simulink model "Threephase_PWM_Inverter"  (R2022b)
settings: Solver=VariableStepAuto  StartTime=0.0  StopTime=2  MaxStep=1e-6
InitFcn:
  | fs=20e3;
  | Ts=1/fs;
  | Udc=700;
  | Cf=20e-6;
  | Rf=0.1;
  | Lf=3e-3;
  | Rg=0.2;
  | Lg=4e-3;
  | wCf=100*pi*Cf;
  | wLf=100*pi*Lf;
  | 
  | Vn=220*sqrt(2);
  | Qn=5000;
  | wn=2*pi*50;
  | Pn=20e3;
  | m=0.01*wn/Pn;
  | kw=1/m;
  | n=1/20*Vn/Qn;
  | J=0.5; %0.2 0.5 0.8
  | D=20;%D=5 10
  | 
  | kp_v=3; %3
  | ki_v=8; %8
  | kp_i=95; %95
  | ki_i=100; %100
libraries: simulink x7, spsabctodq0Lib x6, slpidlib x5, spsThreePhaseSeriesRLCLoadLib x4, spsThreePhaseVIMeasurementLib x4, spsPower3phInstantaneousLib x3, spsThreePhaseBreakerLib x3, spsPLL3phLib x2, spsThreePhaseSeriesRLCBranchLib x2, spsDCVoltageSourceLib x1, spsGroundLib x1, spsUniversalBridgeLib x1
settings Model: Creator=Administrator  LastModifiedBy=Zeren
settings SolverCC: AlgebraicLoopSolver=TrustRegion
settings DataIOCC: ReturnWorkspaceOutputs=off
settings DebuggingCC: UnconnectedInputMsg=warning  UnconnectedOutputMsg=warning  UnconnectedLineMsg=warning  SFMachineParentedDataDiag=warning  ArithmeticOperatorsInVariantConditions=warning
settings ModelReferenceCC: EnableRefExpFcnMdlSchedulingChecks=on
settings SFSimCC: SimUseLocalCustomCode=off  CustomCodeUndefinedFunction=UseInterfaceOnly
settings RTWCC: RTWUseLocalCustomCode=off

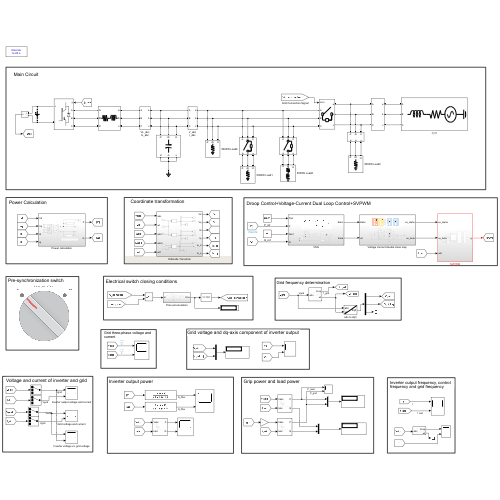
[thumbnail: Simulink's stored preview of the top-level diagram]
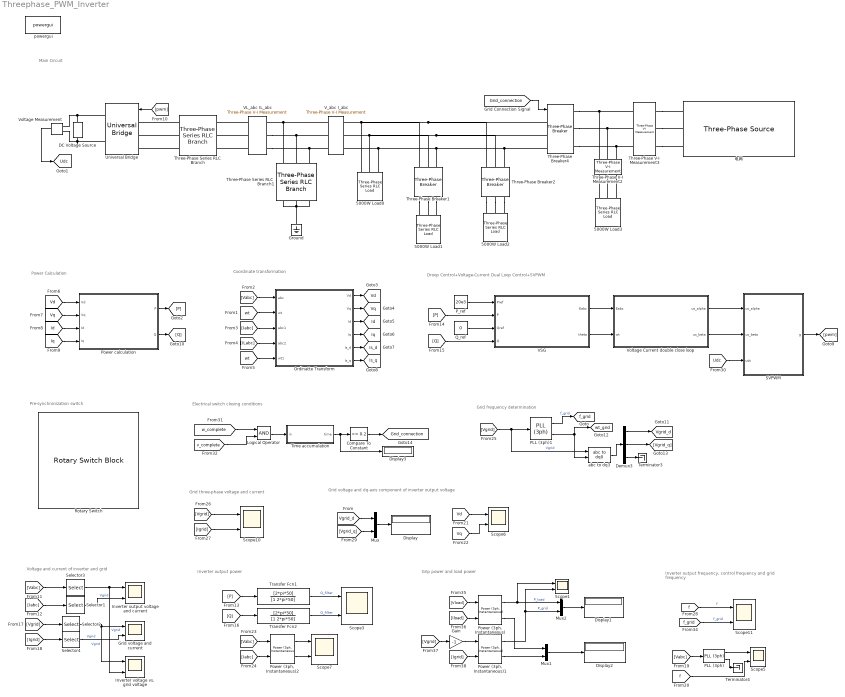
== system Threephase_PWM_Inverter ==
  note: Grid voltage and dq-axis component of inverter output voltage
  note: Grip power and load power
  note: Grid three-phase voltage and current
  note: Voltage and current of inverter and grid
  note: Inverter output frequency, control frequency and grid frequency
  note: Inverter output power
  note: Main Circuit
  note: Grid frequency determination
  note: Power Calculation
  note: Electrical switch closing conditions
  note: Pre-synchronization switch
  note: Coordinate transformation
  note: Droop Control+Voltage-Current Dual Loop Control+SVPWM
  5000W Load0 : spsThreePhaseSeriesRLCLoadLib/Three-Phase Series RLC Load  LConnTagsString=A|B|C  Configuration=Y (grounded)  NominalVoltage=380  Vabc=[1e3 1e3 1e3]  Vabcp=[1e3 1e3 1e3]  NominalFrequency=50  UnbalancedPower=off  ActivePower=5e3  InductivePower=0  CapacitivePower=0  Pabc=[10e3 9e3 11e3]  QLabc=[100 90 110]  QCabc=[100 90 110]  Pabcp=[10e3 9e3 11e3]  QLabcp=[100 90 110]  QCabcp=[100 90 110]  Measurements=None  LoadType=constant Z
  5000W Load1 : spsThreePhaseSeriesRLCLoadLib/Three-Phase Series RLC Load  LConnTagsString=A|B|C  Configuration=Y (grounded)  NominalVoltage=380  Vabc=[1e3 1e3 1e3]  Vabcp=[1e3 1e3 1e3]  NominalFrequency=50  UnbalancedPower=off  ActivePower=5e3  InductivePower=0  CapacitivePower=0  Pabc=[10e3 9e3 11e3]  QLabc=[100 90 110]  QCabc=[100 90 110]  Pabcp=[10e3 9e3 11e3]  QLabcp=[100 90 110]  QCabcp=[100 90 110]  Measurements=None  LoadType=constant Z
  5000W Load2 : spsThreePhaseSeriesRLCLoadLib/Three-Phase Series RLC Load  LConnTagsString=A|B|C  Configuration=Y (grounded)  NominalVoltage=380  Vabc=[1e3 1e3 1e3]  Vabcp=[1e3 1e3 1e3]  NominalFrequency=50  UnbalancedPower=off  ActivePower=5e3  InductivePower=500  CapacitivePower=0  Pabc=[10e3 9e3 11e3]  QLabc=[100 90 110]  QCabc=[100 90 110]  Pabcp=[10e3 9e3 11e3]  QLabcp=[100 90 110]  QCabcp=[100 90 110]  Measurements=None  LoadType=constant Z
  5000W Load3 : spsThreePhaseSeriesRLCLoadLib/Three-Phase Series RLC Load  LConnTagsString=A|B|C  Configuration=Y (grounded)  NominalVoltage=380  Vabc=[1e3 1e3 1e3]  Vabcp=[1e3 1e3 1e3]  NominalFrequency=50  UnbalancedPower=off  ActivePower=5e3  InductivePower=0  CapacitivePower=0  Pabc=[10e3 9e3 11e3]  QLabc=[100 90 110]  QCabc=[100 90 110]  Pabcp=[10e3 9e3 11e3]  QLabcp=[100 90 110]  QCabcp=[100 90 110]  Measurements=None  LoadType=constant Z
  Compare To Constant : simulink/Logic and Bit Operations/Compare To Constant  relop=>=  const=0.2  OutDataTypeStr=boolean
  DC Voltage Source : spsDCVoltageSourceLib/DC Voltage Source  Amplitude=800  Measurements=None
  Demux3 : Demux  Outputs=3
  Display{,1..3} (4 alike) : Display
  Gain : Gain  Gain=-1
  Grid voltage and current : Scope  NumInputPorts=2
  Ground : spsGroundLib/Ground  LConnTagsString=a
  Inverter output voltage and current : Scope  NumInputPorts=2
  Inverter voltage vs. grid voltage : Scope  NumInputPorts=2
  Logical Operator : Logic  AllPortsSameDT=off  OutDataTypeStr=boolean
  Mux : Mux  Inputs=2
  Mux1 : Mux  Inputs=2
  Mux2 : Mux  Inputs=2
  Ordinatte Transform : Subsystem
  PLL (3ph) : spsPLL3phLib/PLL (3ph)  Fmin=45  Par_Init=[0, 50]  ParK=[180, 3200, 1]  TcD=1e-4  MaxRateChangeFreq=12  FilterCutOffFreq=25  Ts=0  AGC=on
  PLL (3ph)1 : spsPLL3phLib/PLL (3ph)  Fmin=45  Par_Init=[0, 50]  ParK=[180, 3200, 1]  TcD=1e-4  MaxRateChangeFreq=12  FilterCutOffFreq=25  Ts=0  AGC=on
  P_ref : Constant  Value=20e3
  "Power (3ph, Instantaneous)" : spsPower3phInstantaneousLib/Power (3ph, Instantaneous)
  "Power (3ph, Instantaneous)1" : spsPower3phInstantaneousLib/Power (3ph, Instantaneous)
  "Power (3ph, Instantaneous)2" : spsPower3phInstantaneousLib/Power (3ph, Instantaneous)
  Power calculation : Subsystem
  Q_ref : Constant  Value=0
  Rotary Switch : RotarySwitchBlock
      settings: Values={{'Off', 'On'}, [0 1]}
  SVPWM : Subsystem
  Scope{1,3,5..7,10..11} (7 alike) : Scope  NumInputPorts=2
  Selector{1..4} (4 alike) : Selector  InputPortWidth=3  IndexOptions=Index vector (dialog)  Indices=[1]  OutputSizes=1
  Terminator3 : Terminator
  Terminator4 : Terminator
  Three-Phase Series RLC Branch : spsThreePhaseSeriesRLCBranchLib/Three-Phase Series RLC Branch  LConnTagsString=A|B|C  RConnTagsString=A|B|C  BranchType=RL  Resistance=1e-4  Inductance=5e-3  Capacitance=1e-6  Measurements=None
  Three-Phase Series RLC Branch1 : spsThreePhaseSeriesRLCBranchLib/Three-Phase Series RLC Branch  LConnTagsString=A|B|C  RConnTagsString=A|B|C  BranchType=C  Resistance=1e-4  Inductance=3e-3  Capacitance=20e-6  Measurements=None
  Three-Phase V-I Measurement2 : spsThreePhaseVIMeasurementLib/Three-Phase V-I Measurement  VoltageMeasurement=phase-to-ground  SetLabelV=on  LabelV=Vload  Vpu=off  VpuLL=off  CurrentMeasurement=yes  SetLabelI=on  LabelI=Iload  Ipu=off  Pbase=100e6  Vbase=500e3  OutputType=Complex  PhasorSimulation=off  PSBequivalent=0
  Three-Phase V-I Measurement3 : spsThreePhaseVIMeasurementLib/Three-Phase V-I Measurement  VoltageMeasurement=phase-to-ground  SetLabelV=on  LabelV=Vgrid  Vpu=off  VpuLL=off  CurrentMeasurement=yes  SetLabelI=on  LabelI=Igrid  Ipu=off  Pbase=100e6  Vbase=500e3  OutputType=Complex  PhasorSimulation=off  PSBequivalent=0
  Three-Phase Breaker1 : spsThreePhaseBreakerLib/Three-Phase Breaker  InitialState=open  SwitchA=on  SwitchB=on  SwitchC=on  SwitchTimes=[0.1]  External=off  BreakerResistance=0.01  SnubberResistance=1e6  SnubberCapacitance=inf  Measurements=None
  Three-Phase Breaker2 : spsThreePhaseBreakerLib/Three-Phase Breaker  InitialState=open  SwitchA=on  SwitchB=on  SwitchC=on  SwitchTimes=[0.15]  External=off  BreakerResistance=0.01  SnubberResistance=1e6  SnubberCapacitance=inf  Measurements=None
  Three-Phase Breaker4 : spsThreePhaseBreakerLib/Three-Phase Breaker  InitialState=open  SwitchA=on  SwitchB=on  SwitchC=on  SwitchTimes=[0.1]  External=on  BreakerResistance=0.01  SnubberResistance=1e6  SnubberCapacitance=inf  Measurements=None
  Time accumulation : Subsystem
  Transfer Fcn1 : TransferFcn  Numerator=[2*pi*50]  Denominator=[1 2*pi*50]
  Transfer Fcn2 : TransferFcn  Numerator=[2*pi*50]  Denominator=[1 2*pi*50]
  Universal Bridge : spsUniversalBridgeLib/Universal Bridge  Arms=3  SnubberResistance=1e5  SnubberCapacitance=inf  Device=IGBT / Diodes  Ron=1e-3  Lon=0  ForwardVoltages="[  0  0  ]"  ForwardVoltage=0  GTOparameters=[ 10e-6 , 20e-6 ]  IGBTparameters=[ 1e-6 , 2e-6 ]  Measurements=None  Measurements_2=None  converterType=Rectifier
  VL_abc IL_abc : spsThreePhaseVIMeasurementLib/Three-Phase V-I Measurement  VoltageMeasurement=no  SetLabelV=off  LabelV=VLabc  Vpu=off  VpuLL=off  CurrentMeasurement=yes  SetLabelI=on  LabelI=ILabc  Ipu=off  Pbase=100e6  Vbase=500e3  OutputType=Complex  PhasorSimulation=off  PSBequivalent=0
  VSG : Subsystem
  V_abc I_abc : spsThreePhaseVIMeasurementLib/Three-Phase V-I Measurement  VoltageMeasurement=phase-to-ground  SetLabelV=on  LabelV=Vabc  Vpu=off  VpuLL=off  CurrentMeasurement=yes  SetLabelI=on  LabelI=Iabc  Ipu=off  Pbase=100e6  Vbase=500e3  OutputType=Complex  PhasorSimulation=off  PSBequivalent=0
  "Voltage Current double close loop " : Subsystem
  Voltage Measurement : spsVoltageMeasurementLib/Voltage Measurement  PhasorSimulation=off  OutputType=Complex  PSBequivalent=0
  abc to dq3 : spsabctodq0Lib/abc to dq0  Alignment=90 degrees behind phase A axis
  powergui : sps_lib/powergui  Priority=1  SimulationMode=Discrete  SampleTime=1e-6  frequency=60  Iterations=50  frequencyindice=0  Pbase=100e6  ErrMax=1e-4  UnitsV=kV  UnitsW=MW  buscounter=0  FunctionMessages=off  echomessages=off  EnableUseOfTLC=off  CurrentSourceSwitches=off  DisableSnubberDevices=off  DisableRonSwitches=off  DisableVfSwitches=off  DisplayEquations=off  AutomaticDiscreteSolvers=off  SolverType=Tustin/Backward Euler (TBE)  Interpol=off  ExternalGateDelay=off  methode=off  Ts=100  x0status=blocks  SPID=on  SwTol=0  HookPort=off  NonlinearTolerance=1e-4  nMaxIteration=100  ContinueOnMaxIteration=off  RestoreLinks=warning  ResistiveCurrentMeasurement=off  Frange=[0:2:500]  Ylog=off  Xlog=on  ShowGrid=off  save=off  variable=ZData  structure=ScopeData2  ZoomFFT=off  StartTime=0.8  cycles=10  DisplayStyle=1  fundamental=50  FreqAxis=off  MaxFrequency=1000  frequencyindicesteady=1  RmsSteady=1  display=off
  电网 : spsThreePhaseSourceLib/Three-Phase Source  InternalConnection=Yg  VoltagePhases=off  Voltage=380  PhaseAngle=20  Voltage_phases=[25e3 25e3 25e3]/sqrt(3)  PhaseAngles_phases=[0 -120 +120]  Frequency=50  NonIdealSource=on  SpecifyImpedance=off  Resistance=1e-4  Inductance=1e-3  ShortCircuitLevel=100e6  BaseVoltage=380  XRratio=7  BusType=swing  Pref=10e3  Qref=0  Prefabc=[10e3, 10e3, 10e3]  Qrefabc=[0, 0, 0]  Qmin=-inf  Qmax=inf
  tag scope: Grid_connection=global, Id=global, Iq=global, Is_d=global, Is_q=global, Udc=global, Vd=global, Vgrid_d=global, Vq=global, f_grid=global, wt_grid=global
  wires:
  Voltage Measurement/1 -> [Udc]
  [pwm] -> Universal Bridge/1
  VSG/1(Eabc) -> "Voltage Current double close loop "/1(Eabc)
  VSG/2(theta) -> "Voltage Current double close loop "/2(wt)
  P_ref/1 -> VSG/1(Pref)
  Q_ref/1 -> VSG/3(Qref)
  [Vd] -> Power calculation/1(Vd)
  [Vq] -> Power calculation/2(Vq)
  [Id] -> Power calculation/3(Id)
  [Iq] -> Power calculation/4(Iq)
  [Vabc] -> Selector3/1
  [Iabc] -> Selector1/1
  Power calculation/1(P) -> [P]
  Power calculation/2(Q) -> [Q]
  [P] -> VSG/2(P)
  [Q] -> VSG/4(Q)
  [Igrid] -> Selector4/1
  [Vgrid] -> Selector2/1
  [Vabc] -> PLL (3ph)/1
  PLL (3ph)/1 -> Scope5/1
  [f] -> Scope5/2
  [Vd] -> Scope6/1
  [Vq] -> Scope6/2
  [Vabc] -> "Power (3ph, Instantaneous)2"/1
  [Iabc] -> "Power (3ph, Instantaneous)2"/2
  "Power (3ph, Instantaneous)2"/1 -> Scope7/1
  "Power (3ph, Instantaneous)2"/2 -> Scope7/2
  [Vgrid] -> PLL (3ph)1/1, abc to dq3/1  "Vgrid"
  PLL (3ph)1/2 -> [wt_grid], abc to dq3/2
  abc to dq3/1 -> Demux3/1
  Demux3/3 -> Terminator3/1
  [Vgrid] -> Scope10/1
  [Igrid] -> Scope10/2
  PLL (3ph)1/1 -> [f_grid]  "f_grid"
  [Udc] -> SVPWM/3(udc)
  Demux3/1 -> [Vgrid_d]
  Demux3/2 -> [Vgrid_q]
  "Voltage Current double close loop "/1(us_alpha) -> SVPWM/1(us_alpha)
  "Voltage Current double close loop "/2(us_beta) -> SVPWM/2(us_beta)
  [w_complete] -> Logical Operator/1
  [v_complete] -> Logical Operator/2
  Logical Operator/1 -> Time accumulation/1(in)
  Compare To Constant/1 -> [Grid_connection]
  [Grid_connection] -> Three-Phase Breaker4/1
  [Vgrid_d] -> Mux/1
  [Vgrid_q] -> Mux/2
  Mux/1 -> Display/1
  [f] -> Scope11/1  "f"
  [f_grid] -> Scope11/2  "f_grid"
  [Vload] -> "Power (3ph, Instantaneous)"/1
  [Iload] -> "Power (3ph, Instantaneous)"/2
  [Igrid] -> "Power (3ph, Instantaneous)1"/2
  [Vgrid] -> Gain/1
  "Power (3ph, Instantaneous)"/1 -> Mux2/1, Scope1/1  "P_load"
  "Power (3ph, Instantaneous)1"/1 -> Mux2/2, Scope1/2  "P_grid"
  "Power (3ph, Instantaneous)1"/2 -> Mux1/2
  Mux1/1 -> Display2/1
  Mux2/1 -> Display1/1
  Time accumulation/1(time) -> Display3/1, Compare To Constant/1
  Selector3/1 -> Inverter output voltage and current/1, Inverter voltage vs. grid voltage/2  "Vgrid"
  Selector1/1 -> Inverter output voltage and current/2  "Vgrid"
  Selector2/1 -> Inverter voltage vs. grid voltage/1, Grid voltage and current/1  "Vgrid"
  Selector4/1 -> Grid voltage and current/2  "Vgrid"
  "Power (3ph, Instantaneous)"/2 -> Mux1/1
  Gain/1 -> "Power (3ph, Instantaneous)1"/1
  PLL (3ph)/2 -> Terminator4/1
  SVPWM/1(g) -> [pwm]
  [Q] -> Transfer Fcn2/1
  Transfer Fcn2/1 -> Scope3/2  "Q_filter"
  [P] -> Transfer Fcn1/1
  Transfer Fcn1/1 -> Scope3/1  "Q_filter"
  [Vabc] -> Ordinatte Transform/1(abc)
  [wt] -> Ordinatte Transform/2(wt)
  [Iabc] -> Ordinatte Transform/3(abc1)
  [ILabc] -> Ordinatte Transform/4(abc2)
  [wt] -> Ordinatte Transform/5(wt1)
  Ordinatte Transform/1(Vd) -> [Vd]
  Ordinatte Transform/2(Vq) -> [Vq]
  Ordinatte Transform/3(Id) -> [Id]
  Ordinatte Transform/4(Iq) -> [Iq]
  Ordinatte Transform/5(Is_d) -> [Is_d]
  Ordinatte Transform/6(Is_q) -> [Is_q]
  connections:
  Universal Bridge/RConn1 -- Voltage Measurement/LConn1 -- DC Voltage Source/RConn1
  DC Voltage Source/LConn1 -- Voltage Measurement/LConn2 -- Universal Bridge/RConn2
  Three-Phase Series RLC Branch/LConn2 -- Universal Bridge/LConn2
  Three-Phase Series RLC Branch/LConn1 -- Universal Bridge/LConn1
  Three-Phase Series RLC Branch/LConn3 -- Universal Bridge/LConn3
  VL_abc IL_abc/LConn2 -- Three-Phase Series RLC Branch/RConn2
  VL_abc IL_abc/LConn1 -- Three-Phase Series RLC Branch/RConn1
  VL_abc IL_abc/LConn3 -- Three-Phase Series RLC Branch/RConn3
  Three-Phase Series RLC Branch1/LConn1 -- V_abc I_abc/LConn1 -- VL_abc IL_abc/RConn1
  VL_abc IL_abc/RConn2 -- V_abc I_abc/LConn2 -- Three-Phase Series RLC Branch1/LConn2
  VL_abc IL_abc/RConn3 -- V_abc I_abc/LConn3 -- Three-Phase Series RLC Branch1/LConn3
  Three-Phase Series RLC Branch1/RConn1 -- Ground/LConn1 -- Three-Phase Series RLC Branch1/RConn2 -- Three-Phase Series RLC Branch1/RConn3
  Three-Phase V-I Measurement2/LConn1 -- Three-Phase Breaker4/RConn1 -- Three-Phase V-I Measurement3/LConn1
  Three-Phase V-I Measurement3/RConn2 -- 电网/RConn2
  Three-Phase V-I Measurement3/RConn1 -- 电网/RConn1
  Three-Phase V-I Measurement3/RConn3 -- 电网/RConn3
  Three-Phase V-I Measurement2/LConn3 -- Three-Phase Breaker4/RConn3 -- Three-Phase V-I Measurement3/LConn3
  Three-Phase V-I Measurement2/RConn2 -- 5000W Load3/LConn2
  Three-Phase V-I Measurement2/RConn3 -- 5000W Load3/LConn3
  Three-Phase V-I Measurement2/RConn1 -- 5000W Load3/LConn1
  Three-Phase V-I Measurement3/LConn2 -- Three-Phase Breaker4/RConn2 -- Three-Phase V-I Measurement2/LConn2
  5000W Load0/LConn1 -- Three-Phase Breaker1/LConn1 -- Three-Phase Breaker2/LConn1 -- Three-Phase Breaker4/LConn1 -- V_abc I_abc/RConn1
  5000W Load0/LConn2 -- Three-Phase Breaker1/LConn2 -- Three-Phase Breaker2/LConn2 -- Three-Phase Breaker4/LConn2 -- V_abc I_abc/RConn2
  Three-Phase Breaker1/RConn2 -- 5000W Load1/LConn2
  Three-Phase Breaker1/RConn3 -- 5000W Load1/LConn3
  Three-Phase Breaker1/RConn1 -- 5000W Load1/LConn1
  Three-Phase Breaker2/RConn1 -- 5000W Load2/LConn1
  Three-Phase Breaker2/RConn2 -- 5000W Load2/LConn2
  Three-Phase Breaker2/RConn3 -- 5000W Load2/LConn3
  Three-Phase Breaker1/LConn3 -- Three-Phase Breaker2/LConn3 -- Three-Phase Breaker4/LConn3 -- 5000W Load0/LConn3 -- V_abc I_abc/RConn3

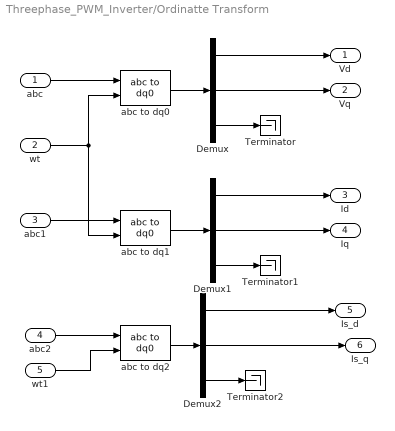
== system Threephase_PWM_Inverter/Ordinatte Transform ==
  abc : Inport
  wt : Inport  Port=2
  abc1 : Inport  Port=3
  abc2 : Inport  Port=4
  wt1 : Inport  Port=5
  Demux : Demux  Outputs=3
  Demux1 : Demux  Outputs=3
  Demux2 : Demux  Outputs=3
  Terminator : Terminator
  Terminator1 : Terminator
  Terminator2 : Terminator
  abc to dq0 : spsabctodq0Lib/abc to dq0  Alignment=90 degrees behind phase A axis
  abc to dq1 : spsabctodq0Lib/abc to dq0  Alignment=90 degrees behind phase A axis
  abc to dq2 : spsabctodq0Lib/abc to dq0  Alignment=90 degrees behind phase A axis
  Vd : Outport
  Vq : Outport  Port=2
  Id : Outport  Port=3
  Iq : Outport  Port=4
  Is_d : Outport  Port=5
  Is_q : Outport  Port=6
  wires:
  wt/1 -> abc to dq0/2, abc to dq1/2
  abc to dq1/1 -> Demux1/1
  Demux1/3 -> Terminator1/1
  Demux/2 -> Vq/1
  abc to dq2/1 -> Demux2/1
  abc1/1 -> abc to dq1/1
  abc to dq0/1 -> Demux/1
  Demux2/3 -> Terminator2/1
  Demux/3 -> Terminator/1
  abc/1 -> abc to dq0/1
  wt1/1 -> abc to dq2/2
  Demux2/1 -> Is_d/1
  Demux/1 -> Vd/1
  Demux1/2 -> Iq/1
  abc2/1 -> abc to dq2/1
  Demux2/2 -> Is_q/1
  Demux1/1 -> Id/1

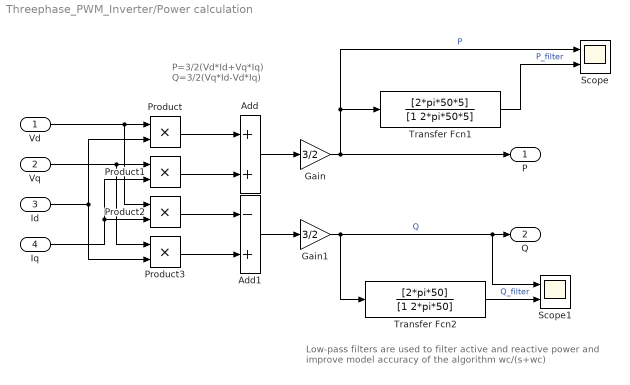
== system Threephase_PWM_Inverter/Power calculation ==
  note: Low-pass filters are used to filter active and reactive power and improve model accuracy of the algorithm wc/(s+wc)
  note: P=3/2(Vd*Id+Vq*Iq)
      |
      | Q=3/2(Vq*Id-Vd*Iq)
  Vd : Inport
  Vq : Inport  Port=2
  Id : Inport  Port=3
  Iq : Inport  Port=4
  Add : Sum
  Add1 : Sum  Inputs=-+
  Gain : Gain  Gain=3/2
  Gain1 : Gain  Gain=3/2
  Product{,1..3} (4 alike) : Product
  Scope : Scope  NumInputPorts=2
  Scope1 : Scope  NumInputPorts=2
  Transfer Fcn1 : TransferFcn  Numerator=[2*pi*50*5]  Denominator=[1 2*pi*50*5]
  Transfer Fcn2 : TransferFcn  Numerator=[2*pi*50]  Denominator=[1 2*pi*50]
  P : Outport  VectorParamsAs1DForOutWhenUnconnected=off
  Q : Outport  Port=2  VectorParamsAs1DForOutWhenUnconnected=off
  wires:
  Add/1 -> Gain/1
  Product/1 -> Add/1
  Product3/1 -> Add1/2
  Add1/1 -> Gain1/1
  Id/1 -> Product3/2, Product/2
  Vq/1 -> Product3/1, Product1/1
  Product1/1 -> Add/2
  Vd/1 -> Product2/1, Product/1
  Product2/1 -> Add1/1
  Gain1/1 -> Scope1/1, Q/1, Transfer Fcn2/1  "Q"
  Iq/1 -> Product2/2, Product1/2
  Gain/1 -> P/1, Scope/1, Transfer Fcn1/1  "P"
  Transfer Fcn2/1 -> Scope1/2  "Q_filter"
  Transfer Fcn1/1 -> Scope/2  "P_filter"

== system Threephase_PWM_Inverter/SVPWM ==
  us_alpha : Inport
  us_beta : Inport  Port=2
  udc : Inport  Port=3
  Constant : Constant  Value=1/fs
  各扇区切换时间 : Subsystem
  开关信号产生 : Subsystem
  扇区位置判断 : Subsystem
  相邻矢量作用时间计算 : Subsystem
  g : Outport  VectorParamsAs1DForOutWhenUnconnected=off
  wires:
  各扇区切换时间/1(Ta) -> 开关信号产生/1(Ta)
  us_beta/1 -> 相邻矢量作用时间计算/2(us_beta), 扇区位置判断/2(us_beta)
  扇区位置判断/1(N(扇区编号)) -> 相邻矢量作用时间计算/5(N), 各扇区切换时间/4(N)
  各扇区切换时间/3(Tc) -> 开关信号产生/3(Tc)
  相邻矢量作用时间计算/1(Tx) -> 各扇区切换时间/2(Tx)
  相邻矢量作用时间计算/2(Ty) -> 各扇区切换时间/3(Ty)
  Constant/1 -> 相邻矢量作用时间计算/3(Ts), 各扇区切换时间/1(Ts)
  各扇区切换时间/2(Tb) -> 开关信号产生/2(Tb)
  开关信号产生/1(g) -> g/1
  us_alpha/1 -> 相邻矢量作用时间计算/1(us_alpha), 扇区位置判断/1(us_alpha)
  udc/1 -> 相邻矢量作用时间计算/4(udc)

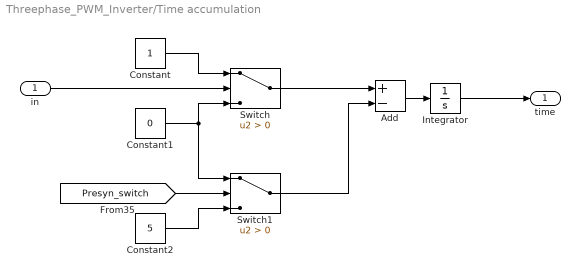
== system Threephase_PWM_Inverter/Time accumulation ==
  in : Inport
  Add : Sum  Inputs=+-
  Constant : Constant
  Constant1 : Constant  Value=0
  Constant2 : Constant  Value=5
  Integrator : Integrator  LimitOutput=on  UpperSaturationLimit=5  LowerSaturationLimit=0
  Switch : Switch  Criteria=u2 > Threshold  SaturateOnIntegerOverflow=off  InputSameDT=off
  Switch1 : Switch  Criteria=u2 > Threshold  SaturateOnIntegerOverflow=off  InputSameDT=off
  time : Outport  VectorParamsAs1DForOutWhenUnconnected=off
  wires:
  in/1 -> Switch/2
  Constant/1 -> Switch/1
  Constant1/1 -> Switch1/1, Switch/3
  Integrator/1 -> time/1
  Add/1 -> Integrator/1
  Switch/1 -> Add/1
  Switch1/1 -> Add/2
  [Presyn_switch] -> Switch1/2
  Constant2/1 -> Switch1/3

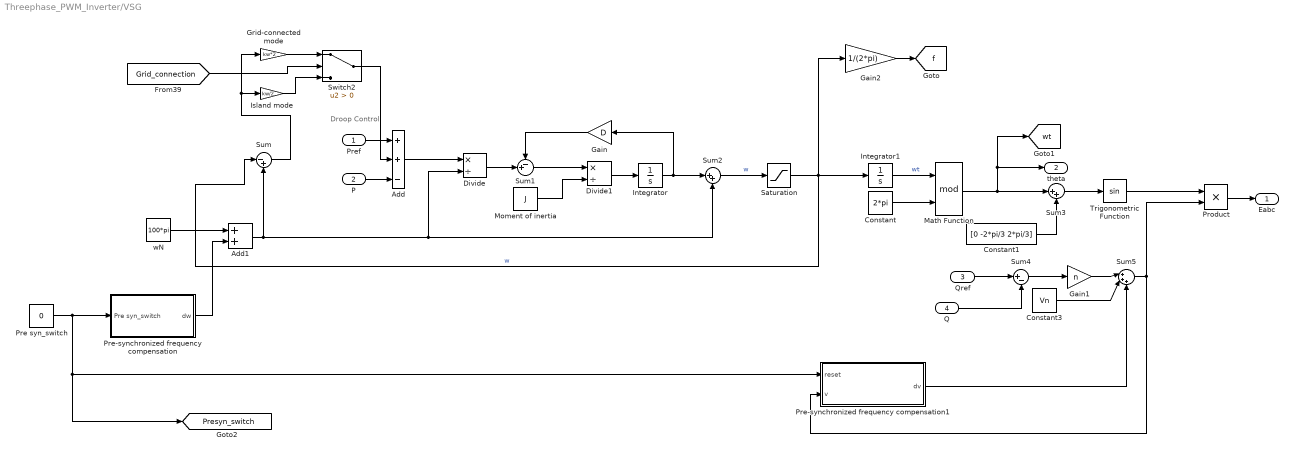
== system Threephase_PWM_Inverter/VSG ==
  note: Droop Control
  Pref : Inport
  P : Inport  Port=2
  Qref : Inport  Port=3
  Q : Inport  Port=4
  Add : Sum  Inputs=++-
  Add1 : Sum
  Constant : Constant  Value=2*pi
  Constant1 : Constant  Value=[0 -2*pi/3 2*pi/3]
  Constant3 : Constant  Value=Vn
  Divide : Product  Inputs=*/
  Divide1 : Product  Inputs=*/
  Gain : Gain  Gain=D
  Gain1 : Gain  Gain=n
  Gain2 : Gain  Gain=1/(2*pi)
  Grid-connected mode : Gain  Gain=kw*2
  Integrator : Integrator
  Integrator1 : Integrator
  Island mode : Gain  Gain=kw/2
  Math Function : Math  Operator=mod  SignedPower=on
  Moment of inertia : Constant  Value=J
  Pre syn_switch : Constant  Value=0
  Pre-synchronized frequency compensation : Subsystem
  Pre-synchronized frequency compensation1 : Subsystem
  Product : Product
  Saturation : Saturate  UpperLimit=2*pi*50.5  LowerLimit=2*pi*49.5
  Sum : Sum  Inputs=|-+
  Sum1 : Sum  Inputs=-+|
  Sum2 : Sum  Inputs=|++
  Sum3 : Sum  Inputs=|++
  Sum4 : Sum  Inputs=|+-
  Sum5 : Sum  Inputs=|+++
  Switch2 : Switch  Criteria=u2 > Threshold  SaturateOnIntegerOverflow=off  InputSameDT=off
  Trigonometric Function : Trigonometry
  wN : Constant  Value=100*pi
  Eabc : Outport  VectorParamsAs1DForOutWhenUnconnected=off
  theta : Outport  Port=2  VectorParamsAs1DForOutWhenUnconnected=off
  tag scope: Presyn_switch=global, f=global, wt=global
  wires:
  Sum/1 -> Island mode/1, Grid-connected mode/1
  Switch2/1 -> Add/2
  Pref/1 -> Add/1
  P/1 -> Add/3
  Add/1 -> Divide/1
  Divide/1 -> Sum1/2
  Sum1/1 -> Divide1/1
  Moment of inertia/1 -> Divide1/2
  Divide1/1 -> Integrator/1
  Integrator/1 -> Sum2/1, Gain/1
  Gain/1 -> Sum1/1
  Integrator1/1 -> Math Function/1  "wt"
  Constant/1 -> Math Function/2
  Math Function/1 -> Sum3/1, theta/1, [wt]
  Constant1/1 -> Sum3/2
  Sum3/1 -> Trigonometric Function/1
  Trigonometric Function/1 -> Product/1
  Qref/1 -> Sum4/1
  Q/1 -> Sum4/2
  Sum4/1 -> Gain1/1
  Gain1/1 -> Sum5/1
  Constant3/1 -> Sum5/2
  Product/1 -> Eabc/1
  Gain2/1 -> [f]
  Sum5/1 -> Product/2, Pre-synchronized frequency compensation1/2(v)
  Pre-synchronized frequency compensation1/1(dv) -> Sum5/3
  Pre syn_switch/1 -> Pre-synchronized frequency compensation1/1(reset), [Presyn_switch], Pre-synchronized frequency compensation/1(Pre syn_switch)
  Saturation/1 -> Gain2/1, Sum/1, Integrator1/1  "w"
  Sum2/1 -> Saturation/1  "w"
  wN/1 -> Add1/1
  Add1/1 -> Divide/2, Sum2/2, Sum/2
  Pre-synchronized frequency compensation/1(dw) -> Add1/2
  [Grid_connection] -> Switch2/2
  Grid-connected mode/1 -> Switch2/1
  Island mode/1 -> Switch2/3

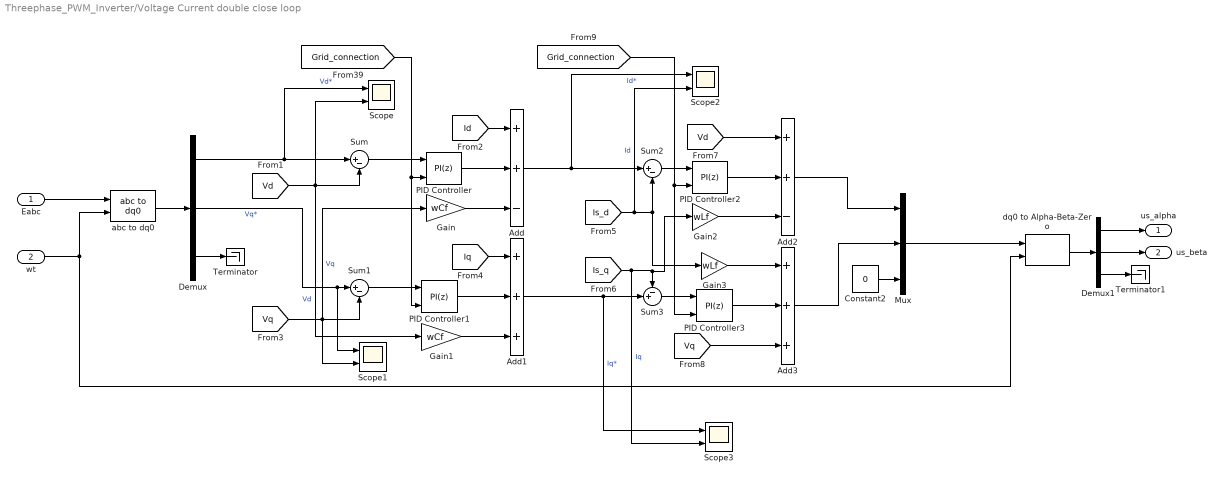
== system Threephase_PWM_Inverter/Voltage Current double close loop  ==
  Eabc : Inport
  wt : Inport  Port=2
  Add : Sum  Inputs=++-
  Add1 : Sum  Inputs=+++
  Add2 : Sum  Inputs=++-
  Add3 : Sum  Inputs=+++
  Constant2 : Constant  Value=0
  Demux : Demux  Outputs=3
  Demux1 : Demux  Outputs=3
  Gain : Gain  Gain=wCf
  Gain1 : Gain  Gain=wCf
  Gain2 : Gain  Gain=wLf
  Gain3 : Gain  Gain=wLf
  Mux : Mux  Inputs=3
  PID Controller : slpidlib/PID Controller  Controller=PI  Form=Parallel  TimeDomain=Discrete-time  UseExternalTs=off  SampleTime=-1  IntegratorMethod=Forward Euler  FilterMethod=Forward Euler  ControllerParametersSource=internal  P=kp_v  I=ki_v  UseKiTs=off  D=0  N=100  UseFilter=on  TunerSelectOption=Transfer Function Based (PID Tuner App)  InitialConditionSource=internal  InitialConditionForIntegrator=0  InitialConditionForFilter=0  DifferentiatorICPrevScaledInput=0  ExternalReset=either  TrackingMode=off  Kt=1  LimitOutput=off  SatLimitsSource=internal  UpperSaturationLimit=inf  LowerSaturationLimit=-inf  LinearizeAsGain=on  AntiWindupMode=none  Kb=1  LimitIntegrator=off  UpperIntegratorSaturationLimit=inf  LowerIntegratorSaturationLimit=-inf  POutMin=[]  POutMax=[]  IOutMin=[]  IOutMax=[]  DOutMin=[]  DOutMax=[]  NOutMin=[]  NOutMax=[]  SumOutMin=[]  SumOutMax=[]  SaturationOutMin=[]  SaturationOutMax=[]  PParamMin=[]  PParamMax=[]  IParamMin=[]  IParamMax=[]  DParamMin=[]  DParamMax=[]  NParamMin=[]  NParamMax=[]  KbParamMin=[]  KbParamMax=[]  KtParamMin=[]  KtParamMax=[]  KbOutMin=[]  KbOutMax=[]  KtOutMin=[]  KtOutMax=[]  IntegratorOutMin=[]  IntegratorOutMax=[]  FilterOutMin=[]  FilterOutMax=[]  SumI1OutMin=[]  SumI1OutMax=[]  SumI2OutMin=[]  SumI2OutMax=[]  SumI3OutMin=[]  SumI3OutMax=[]  SumI4OutMin=[]  SumI4OutMax=[]  SumDOutMin=[]  SumDOutMax=[]  DifferentiatorOutMin=[]  DifferentiatorOutMax=[]  FilterDiffOutCoefMin=[]  FilterDiffOutCoefMax=[]  ReciprocalOutMin=[]  ReciprocalOutMax=[]  SumDenOutMin=[]  SumDenOutMax=[]  SumNumOutMin=[]  SumNumOutMax=[]  DivideOutMin=[]  DivideOutMax=[]  UdiffTsProdOutMin=[]  UdiffTsProdOutMax=[]  NTsProdOutMin=[]  NTsProdOutMax=[]  UintegralTsProdOutMin=[]  UintegralTsProdOutMax=[]  UngainTsProdOutMin=[]  UngainTsProdOutMax=[]  ClampingZeroOutDataTypeStr=Inherit: Inherit via back propagation  ClampingZeroOutMin=[]  ClampingZeroOutMax=[]  FilterDenConstantOutDataTypeStr=Inherit: Inherit via back propagation  FilterDenConstantOutMin=[]  FilterDenConstantOutMax=[]  PCopyOutDataTypeStr=Inherit: Inherit via back propagation  PCopyOutMin=[]  PCopyOutMax=[]  NCopyOutDataTypeStr=Inherit: Inherit via back propagation  NCopyOutMin=[]  NCopyOutMax=[]  IntegratorContinuousStateAttributes=''  IntegratorStateMustResolveToSignalObject=off  IntegratorRTWStateStorageClass=Auto  FilterContinuousStateAttributes=''  FilterStateMustResolveToSignalObject=off  FilterRTWStateStorageClass=Auto  ParallelPVariant=InternalParameters  IdealPVariant=Disabled  IVariant=InternalParameters  DVariant=Disabled  IntegratorVariant=Discrete  SatVariant=Disabled  AWVariant=Passthrough  PCopyVariant=Disabled  TRVariant=Disabled  FdbkBlocksVariant=Forward  IdealPFdbkVariant=Disabled  SatFdbkVariant=Disabled  DerivativeFilterVariant=Disabled  NVariant=Disabled  NCopyVariant=Disabled_SignalSpec  FilterICVariant=Disabled  IntegratorICVariant=InternalICs  ExternalResetVariant=ExternalReset  TRSumVariant=Passthrough  SumFdbkVariant=Disabled  SumVariant=Sum_PI  TsampFilterVariant=InternalTs  TsampNgainVariant=Passthrough  TsampIntegralVariant=Passthrough  ExternalSaturationOutDataTypeStr=Inherit: Same as second input
  PID Controller1 : slpidlib/PID Controller  Controller=PI  Form=Parallel  TimeDomain=Discrete-time  UseExternalTs=off  SampleTime=-1  IntegratorMethod=Forward Euler  FilterMethod=Forward Euler  ControllerParametersSource=internal  P=kp_v  I=ki_v  UseKiTs=off  D=0  N=100  UseFilter=on  TunerSelectOption=Transfer Function Based (PID Tuner App)  InitialConditionSource=internal  InitialConditionForIntegrator=0  InitialConditionForFilter=0  DifferentiatorICPrevScaledInput=0  ExternalReset=either  TrackingMode=off  Kt=1  LimitOutput=off  SatLimitsSource=internal  UpperSaturationLimit=inf  LowerSaturationLimit=-inf  LinearizeAsGain=on  AntiWindupMode=none  Kb=1  LimitIntegrator=off  UpperIntegratorSaturationLimit=inf  LowerIntegratorSaturationLimit=-inf  POutMin=[]  POutMax=[]  IOutMin=[]  IOutMax=[]  DOutMin=[]  DOutMax=[]  NOutMin=[]  NOutMax=[]  SumOutMin=[]  SumOutMax=[]  SaturationOutMin=[]  SaturationOutMax=[]  PParamMin=[]  PParamMax=[]  IParamMin=[]  IParamMax=[]  DParamMin=[]  DParamMax=[]  NParamMin=[]  NParamMax=[]  KbParamMin=[]  KbParamMax=[]  KtParamMin=[]  KtParamMax=[]  KbOutMin=[]  KbOutMax=[]  KtOutMin=[]  KtOutMax=[]  IntegratorOutMin=[]  IntegratorOutMax=[]  FilterOutMin=[]  FilterOutMax=[]  SumI1OutMin=[]  SumI1OutMax=[]  SumI2OutMin=[]  SumI2OutMax=[]  SumI3OutMin=[]  SumI3OutMax=[]  SumI4OutMin=[]  SumI4OutMax=[]  SumDOutMin=[]  SumDOutMax=[]  DifferentiatorOutMin=[]  DifferentiatorOutMax=[]  FilterDiffOutCoefMin=[]  FilterDiffOutCoefMax=[]  ReciprocalOutMin=[]  ReciprocalOutMax=[]  SumDenOutMin=[]  SumDenOutMax=[]  SumNumOutMin=[]  SumNumOutMax=[]  DivideOutMin=[]  DivideOutMax=[]  UdiffTsProdOutMin=[]  UdiffTsProdOutMax=[]  NTsProdOutMin=[]  NTsProdOutMax=[]  UintegralTsProdOutMin=[]  UintegralTsProdOutMax=[]  UngainTsProdOutMin=[]  UngainTsProdOutMax=[]  ClampingZeroOutDataTypeStr=Inherit: Inherit via back propagation  ClampingZeroOutMin=[]  ClampingZeroOutMax=[]  FilterDenConstantOutDataTypeStr=Inherit: Inherit via back propagation  FilterDenConstantOutMin=[]  FilterDenConstantOutMax=[]  PCopyOutDataTypeStr=Inherit: Inherit via back propagation  PCopyOutMin=[]  PCopyOutMax=[]  NCopyOutDataTypeStr=Inherit: Inherit via back propagation  NCopyOutMin=[]  NCopyOutMax=[]  IntegratorContinuousStateAttributes=''  IntegratorStateMustResolveToSignalObject=off  IntegratorRTWStateStorageClass=Auto  FilterContinuousStateAttributes=''  FilterStateMustResolveToSignalObject=off  FilterRTWStateStorageClass=Auto  ParallelPVariant=InternalParameters  IdealPVariant=Disabled  IVariant=InternalParameters  DVariant=Disabled  IntegratorVariant=Discrete  SatVariant=Disabled  AWVariant=Passthrough  PCopyVariant=Disabled  TRVariant=Disabled  FdbkBlocksVariant=Forward  IdealPFdbkVariant=Disabled  SatFdbkVariant=Disabled  DerivativeFilterVariant=Disabled  NVariant=Disabled  NCopyVariant=Disabled_SignalSpec  FilterICVariant=Disabled  IntegratorICVariant=InternalICs  ExternalResetVariant=ExternalReset  TRSumVariant=Passthrough  SumFdbkVariant=Disabled  SumVariant=Sum_PI  TsampFilterVariant=InternalTs  TsampNgainVariant=Passthrough  TsampIntegralVariant=Passthrough  ExternalSaturationOutDataTypeStr=Inherit: Same as second input
  PID Controller2 : slpidlib/PID Controller  Controller=PI  Form=Parallel  TimeDomain=Discrete-time  UseExternalTs=off  SampleTime=-1  IntegratorMethod=Forward Euler  FilterMethod=Forward Euler  ControllerParametersSource=internal  P=kp_i  I=ki_i  UseKiTs=off  D=0  N=100  UseFilter=on  TunerSelectOption=Transfer Function Based (PID Tuner App)  InitialConditionSource=internal  InitialConditionForIntegrator=0  InitialConditionForFilter=0  DifferentiatorICPrevScaledInput=0  ExternalReset=either  TrackingMode=off  Kt=1  LimitOutput=off  SatLimitsSource=internal  UpperSaturationLimit=inf  LowerSaturationLimit=-inf  LinearizeAsGain=on  AntiWindupMode=none  Kb=1  LimitIntegrator=off  UpperIntegratorSaturationLimit=inf  LowerIntegratorSaturationLimit=-inf  POutMin=[]  POutMax=[]  IOutMin=[]  IOutMax=[]  DOutMin=[]  DOutMax=[]  NOutMin=[]  NOutMax=[]  SumOutMin=[]  SumOutMax=[]  SaturationOutMin=[]  SaturationOutMax=[]  PParamMin=[]  PParamMax=[]  IParamMin=[]  IParamMax=[]  DParamMin=[]  DParamMax=[]  NParamMin=[]  NParamMax=[]  KbParamMin=[]  KbParamMax=[]  KtParamMin=[]  KtParamMax=[]  KbOutMin=[]  KbOutMax=[]  KtOutMin=[]  KtOutMax=[]  IntegratorOutMin=[]  IntegratorOutMax=[]  FilterOutMin=[]  FilterOutMax=[]  SumI1OutMin=[]  SumI1OutMax=[]  SumI2OutMin=[]  SumI2OutMax=[]  SumI3OutMin=[]  SumI3OutMax=[]  SumI4OutMin=[]  SumI4OutMax=[]  SumDOutMin=[]  SumDOutMax=[]  DifferentiatorOutMin=[]  DifferentiatorOutMax=[]  FilterDiffOutCoefMin=[]  FilterDiffOutCoefMax=[]  ReciprocalOutMin=[]  ReciprocalOutMax=[]  SumDenOutMin=[]  SumDenOutMax=[]  SumNumOutMin=[]  SumNumOutMax=[]  DivideOutMin=[]  DivideOutMax=[]  UdiffTsProdOutMin=[]  UdiffTsProdOutMax=[]  NTsProdOutMin=[]  NTsProdOutMax=[]  UintegralTsProdOutMin=[]  UintegralTsProdOutMax=[]  UngainTsProdOutMin=[]  UngainTsProdOutMax=[]  ClampingZeroOutDataTypeStr=Inherit: Inherit via back propagation  ClampingZeroOutMin=[]  ClampingZeroOutMax=[]  FilterDenConstantOutDataTypeStr=Inherit: Inherit via back propagation  FilterDenConstantOutMin=[]  FilterDenConstantOutMax=[]  PCopyOutDataTypeStr=Inherit: Inherit via back propagation  PCopyOutMin=[]  PCopyOutMax=[]  NCopyOutDataTypeStr=Inherit: Inherit via back propagation  NCopyOutMin=[]  NCopyOutMax=[]  IntegratorContinuousStateAttributes=''  IntegratorStateMustResolveToSignalObject=off  IntegratorRTWStateStorageClass=Auto  FilterContinuousStateAttributes=''  FilterStateMustResolveToSignalObject=off  FilterRTWStateStorageClass=Auto  ParallelPVariant=InternalParameters  IdealPVariant=Disabled  IVariant=InternalParameters  DVariant=Disabled  IntegratorVariant=Discrete  SatVariant=Disabled  AWVariant=Passthrough  PCopyVariant=Disabled  TRVariant=Disabled  FdbkBlocksVariant=Forward  IdealPFdbkVariant=Disabled  SatFdbkVariant=Disabled  DerivativeFilterVariant=Disabled  NVariant=Disabled  NCopyVariant=Disabled_SignalSpec  FilterICVariant=Disabled  IntegratorICVariant=InternalICs  ExternalResetVariant=ExternalReset  TRSumVariant=Passthrough  SumFdbkVariant=Disabled  SumVariant=Sum_PI  TsampFilterVariant=InternalTs  TsampNgainVariant=Passthrough  TsampIntegralVariant=Passthrough  ExternalSaturationOutDataTypeStr=Inherit: Same as second input
  PID Controller3 : slpidlib/PID Controller  Controller=PI  Form=Parallel  TimeDomain=Discrete-time  UseExternalTs=off  SampleTime=-1  IntegratorMethod=Forward Euler  FilterMethod=Forward Euler  ControllerParametersSource=internal  P=kp_i  I=ki_i  UseKiTs=off  D=0  N=100  UseFilter=on  TunerSelectOption=Transfer Function Based (PID Tuner App)  InitialConditionSource=internal  InitialConditionForIntegrator=0  InitialConditionForFilter=0  DifferentiatorICPrevScaledInput=0  ExternalReset=either  TrackingMode=off  Kt=1  LimitOutput=off  SatLimitsSource=internal  UpperSaturationLimit=inf  LowerSaturationLimit=-inf  LinearizeAsGain=on  AntiWindupMode=none  Kb=1  LimitIntegrator=off  UpperIntegratorSaturationLimit=inf  LowerIntegratorSaturationLimit=-inf  POutMin=[]  POutMax=[]  IOutMin=[]  IOutMax=[]  DOutMin=[]  DOutMax=[]  NOutMin=[]  NOutMax=[]  SumOutMin=[]  SumOutMax=[]  SaturationOutMin=[]  SaturationOutMax=[]  PParamMin=[]  PParamMax=[]  IParamMin=[]  IParamMax=[]  DParamMin=[]  DParamMax=[]  NParamMin=[]  NParamMax=[]  KbParamMin=[]  KbParamMax=[]  KtParamMin=[]  KtParamMax=[]  KbOutMin=[]  KbOutMax=[]  KtOutMin=[]  KtOutMax=[]  IntegratorOutMin=[]  IntegratorOutMax=[]  FilterOutMin=[]  FilterOutMax=[]  SumI1OutMin=[]  SumI1OutMax=[]  SumI2OutMin=[]  SumI2OutMax=[]  SumI3OutMin=[]  SumI3OutMax=[]  SumI4OutMin=[]  SumI4OutMax=[]  SumDOutMin=[]  SumDOutMax=[]  DifferentiatorOutMin=[]  DifferentiatorOutMax=[]  FilterDiffOutCoefMin=[]  FilterDiffOutCoefMax=[]  ReciprocalOutMin=[]  ReciprocalOutMax=[]  SumDenOutMin=[]  SumDenOutMax=[]  SumNumOutMin=[]  SumNumOutMax=[]  DivideOutMin=[]  DivideOutMax=[]  UdiffTsProdOutMin=[]  UdiffTsProdOutMax=[]  NTsProdOutMin=[]  NTsProdOutMax=[]  UintegralTsProdOutMin=[]  UintegralTsProdOutMax=[]  UngainTsProdOutMin=[]  UngainTsProdOutMax=[]  ClampingZeroOutDataTypeStr=Inherit: Inherit via back propagation  ClampingZeroOutMin=[]  ClampingZeroOutMax=[]  FilterDenConstantOutDataTypeStr=Inherit: Inherit via back propagation  FilterDenConstantOutMin=[]  FilterDenConstantOutMax=[]  PCopyOutDataTypeStr=Inherit: Inherit via back propagation  PCopyOutMin=[]  PCopyOutMax=[]  NCopyOutDataTypeStr=Inherit: Inherit via back propagation  NCopyOutMin=[]  NCopyOutMax=[]  IntegratorContinuousStateAttributes=''  IntegratorStateMustResolveToSignalObject=off  IntegratorRTWStateStorageClass=Auto  FilterContinuousStateAttributes=''  FilterStateMustResolveToSignalObject=off  FilterRTWStateStorageClass=Auto  ParallelPVariant=InternalParameters  IdealPVariant=Disabled  IVariant=InternalParameters  DVariant=Disabled  IntegratorVariant=Discrete  SatVariant=Disabled  AWVariant=Passthrough  PCopyVariant=Disabled  TRVariant=Disabled  FdbkBlocksVariant=Forward  IdealPFdbkVariant=Disabled  SatFdbkVariant=Disabled  DerivativeFilterVariant=Disabled  NVariant=Disabled  NCopyVariant=Disabled_SignalSpec  FilterICVariant=Disabled  IntegratorICVariant=InternalICs  ExternalResetVariant=ExternalReset  TRSumVariant=Passthrough  SumFdbkVariant=Disabled  SumVariant=Sum_PI  TsampFilterVariant=InternalTs  TsampNgainVariant=Passthrough  TsampIntegralVariant=Passthrough  ExternalSaturationOutDataTypeStr=Inherit: Same as second input
  Scope{,1..3} (4 alike) : Scope  NumInputPorts=2
  Sum : Sum  Inputs=|+-
  Sum1 : Sum  Inputs=|+-
  Sum2 : Sum  Inputs=|+-
  Sum3 : Sum  Inputs=-+|
  Terminator : Terminator
  Terminator1 : Terminator
  abc to dq0 : spsabctodq0Lib/abc to dq0  Alignment=90 degrees behind phase A axis
  dq0 to Alpha-Beta-Zero : spsdq0toAlphaBetaZeroLib/dq0 to Alpha-Beta-Zero  Alignment=90 degrees behind phase A axis
  us_alpha : Outport  VectorParamsAs1DForOutWhenUnconnected=off
  us_beta : Outport  Port=2  VectorParamsAs1DForOutWhenUnconnected=off
  wires:
  wt/1 -> abc to dq0/2, dq0 to Alpha-Beta-Zero/2
  PID Controller3/1 -> Add3/2
  Gain/1 -> Add/3
  [Is_q] -> Scope3/2, Gain2/1, Sum3/1  "Iq"
  Sum2/1 -> PID Controller2/1
  Demux/3 -> Terminator/1
  Eabc/1 -> abc to dq0/1
  Demux/1 -> Scope/1, Sum/1  "Vd*"
  Sum3/1 -> PID Controller3/1
  [Vd] -> Add2/1
  [Vq] -> Scope1/2, Gain/1, Sum1/2  "Vq"
  abc to dq0/1 -> Demux/1
  Constant2/1 -> Mux/3
  Demux1/3 -> Terminator1/1
  [Is_d] -> Scope2/2, Gain3/1, Sum2/2  "Id"
  Mux/1 -> dq0 to Alpha-Beta-Zero/1
  Demux/2 -> Scope1/1, Sum1/1  "Vq*"
  [Vd] -> Scope/2, Gain1/1, Sum/2  "Vd"
  Gain3/1 -> Add3/1
  PID Controller2/1 -> Add2/2
  [Vq] -> Add3/3
  Sum1/1 -> PID Controller1/1
  Gain1/1 -> Add1/3
  Add3/1 -> Mux/2
  [Iq] -> Add1/1
  PID Controller1/1 -> Add1/2
  Gain2/1 -> Add2/3
  PID Controller/1 -> Add/2
  [Id] -> Add/1
  dq0 to Alpha-Beta-Zero/1 -> Demux1/1
  Sum/1 -> PID Controller/1
  Demux1/1 -> us_alpha/1
  Demux1/2 -> us_beta/1
  Add1/1 -> Scope3/1, Sum3/2  "Iq*"
  Add/1 -> Scope2/1, Sum2/1  "Id*"
  [Grid_connection] -> PID Controller1/2, PID Controller/2
  [Grid_connection] -> PID Controller3/2, PID Controller2/2
  Add2/1 -> Mux/1

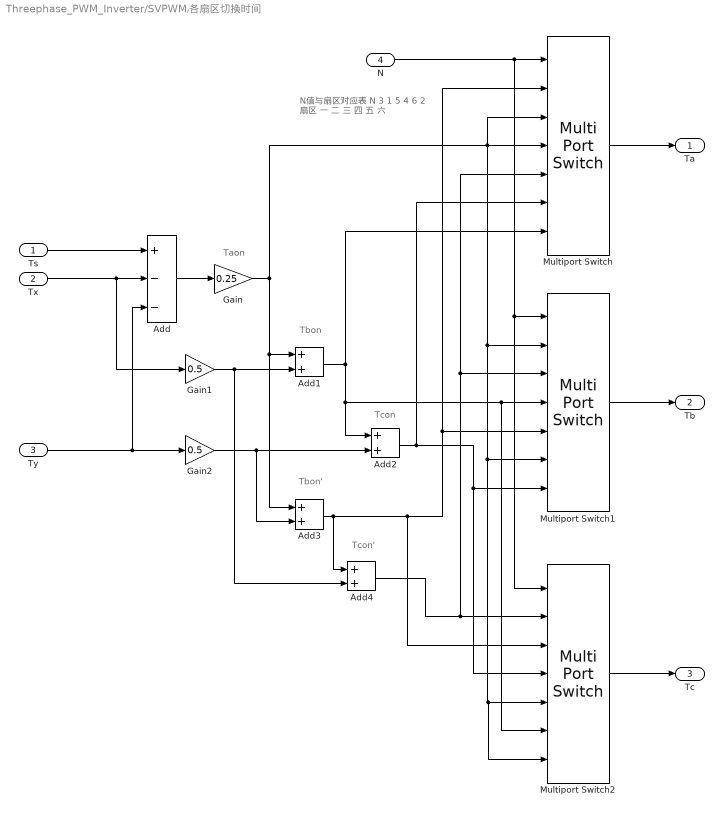
== system Threephase_PWM_Inverter/SVPWM/各扇区切换时间 ==
  note: Tcon'
  note: Tbon'
  note: Tcon
  note: Tbon
  note: Taon
  note: N值与扇区对应表
      | N         3    1    5    4    6    2
      | 扇区    一  二  三  四  五   六
  Ts : Inport
  Tx : Inport  Port=2
  Ty : Inport  Port=3
  N : Inport  Port=4
  Add : Sum  Inputs=+--
  Add{1..4} (4 alike) : Sum
  Gain : Gain  Gain=0.25
  Gain1 : Gain  Gain=0.5
  Gain2 : Gain  Gain=0.5
  Multiport Switch : MultiPortSwitch  Inputs=6  SaturateOnIntegerOverflow=off  InputSameDT=off
  Multiport Switch1 : MultiPortSwitch  Inputs=6  SaturateOnIntegerOverflow=off  InputSameDT=off
  Multiport Switch2 : MultiPortSwitch  Inputs=6  SaturateOnIntegerOverflow=off  InputSameDT=off
  Ta : Outport  VectorParamsAs1DForOutWhenUnconnected=off
  Tb : Outport  Port=2  VectorParamsAs1DForOutWhenUnconnected=off
  Tc : Outport  Port=3  VectorParamsAs1DForOutWhenUnconnected=off
  wires:
  Ty/1 -> Add/3, Gain2/1
  Gain2/1 -> Add3/2, Add2/2
  Add/1 -> Gain/1
  Add2/1 -> Multiport Switch/6, Multiport Switch1/7, Multiport Switch2/4
  Tx/1 -> Gain1/1, Add/2
  Add1/1 -> Multiport Switch/7, Multiport Switch2/6, Multiport Switch1/4, Add2/1
  Ts/1 -> Add/1
  Gain1/1 -> Add4/2, Add1/2
  Multiport Switch/1 -> Ta/1
  Multiport Switch1/1 -> Tb/1
  N/1 -> Multiport Switch2/1, Multiport Switch1/1, Multiport Switch/1
  Multiport Switch2/1 -> Tc/1
  Add3/1 -> Add4/1, Multiport Switch2/3, Multiport Switch1/5, Multiport Switch/2
  Add4/1 -> Multiport Switch1/3, Multiport Switch/5, Multiport Switch2/2
  Gain/1 -> Multiport Switch/3, Multiport Switch1/2, Multiport Switch2/5, Multiport Switch2/7, Multiport Switch1/6, Multiport Switch/4, Add1/1, Add3/1

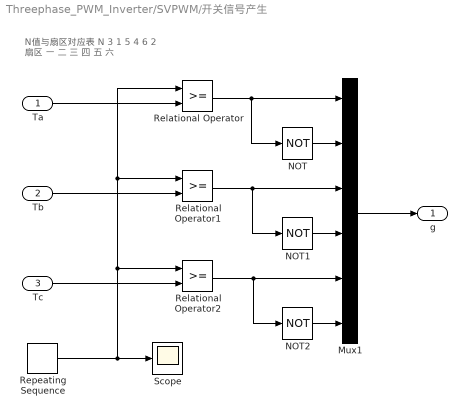
== system Threephase_PWM_Inverter/SVPWM/开关信号产生 ==
  note: N值与扇区对应表
      | N         3    1    5    4    6    2
      | 扇区    一  二  三  四  五   六
  Ta : Inport
  Tb : Inport  Port=2
  Tc : Inport  Port=3
  Mux1 : Mux  Inputs=6
  NOT : Logic  Operator=NOT  IconShape=distinctive  AllPortsSameDT=off  OutDataTypeStr=boolean
  NOT1 : Logic  Operator=NOT  IconShape=distinctive  AllPortsSameDT=off  OutDataTypeStr=boolean
  NOT2 : Logic  Operator=NOT  IconShape=distinctive  AllPortsSameDT=off  OutDataTypeStr=boolean
  Relational Operator : RelationalOperator  OutDataTypeStr=boolean  RndMeth=Simplest  InputSameDT=off
  Relational Operator1 : RelationalOperator  OutDataTypeStr=boolean  RndMeth=Simplest  InputSameDT=off
  Relational Operator2 : RelationalOperator  OutDataTypeStr=boolean  RndMeth=Simplest  InputSameDT=off
  Repeating Sequence : simulink/Sources/Repeating Sequence  rep_seq_t=[0 1/fs/2 1/fs]  rep_seq_y=[0 1/fs/2 0]
  Scope : Scope
  g : Outport  VectorParamsAs1DForOutWhenUnconnected=off
  wires:
  Mux1/1 -> g/1
  Tc/1 -> Relational Operator2/2
  Relational Operator2/1 -> NOT2/1, Mux1/5
  Repeating Sequence/1 -> Scope/1, Relational Operator/1, Relational Operator1/1, Relational Operator2/1
  Tb/1 -> Relational Operator1/2
  NOT2/1 -> Mux1/6
  Ta/1 -> Relational Operator/2
  NOT1/1 -> Mux1/4
  NOT/1 -> Mux1/2
  Relational Operator1/1 -> Mux1/3, NOT1/1
  Relational Operator/1 -> Mux1/1, NOT/1

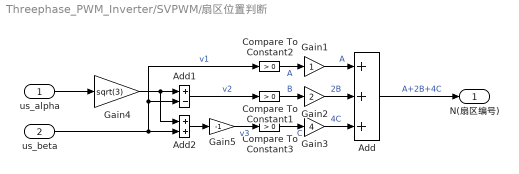
== system Threephase_PWM_Inverter/SVPWM/扇区位置判断 ==
  us_alpha : Inport
  us_beta : Inport  Port=2
  Add : Sum  Inputs=+++
  Add1 : Sum  Inputs=+-
  Add2 : Sum
  Compare To Constant1 : simulink/Logic and Bit Operations/Compare To Constant  relop=>  const=0  OutDataTypeStr=boolean
  Compare To Constant2 : simulink/Logic and Bit Operations/Compare To Constant  relop=>  const=0  OutDataTypeStr=boolean
  Compare To Constant3 : simulink/Logic and Bit Operations/Compare To Constant  relop=>  const=0  OutDataTypeStr=boolean
  Gain1 : Gain
  Gain2 : Gain  Gain=2
  Gain3 : Gain  Gain=4
  Gain4 : Gain  Gain=sqrt(3)
  Gain5 : Gain  Gain=-1
  N(扇区编号) : Outport  VectorParamsAs1DForOutWhenUnconnected=off
  wires:
  Add1/1 -> Compare To Constant1/1  "v2"
  Gain2/1 -> Add/2  "2B"
  Add2/1 -> Gain5/1
  Gain4/1 -> Add2/1, Add1/1
  Gain5/1 -> Compare To Constant3/1  "v3"
  Gain1/1 -> Add/1  "A"
  Compare To Constant1/1 -> Gain2/1  "B"
  Compare To Constant2/1 -> Gain1/1  "A"
  Gain3/1 -> Add/3  "4C"
  us_beta/1 -> Add2/2, Add1/2, Compare To Constant2/1  "v1"
  us_alpha/1 -> Gain4/1
  Compare To Constant3/1 -> Gain3/1  "C"
  Add/1 -> N(扇区编号)/1  "A+2B+4C"

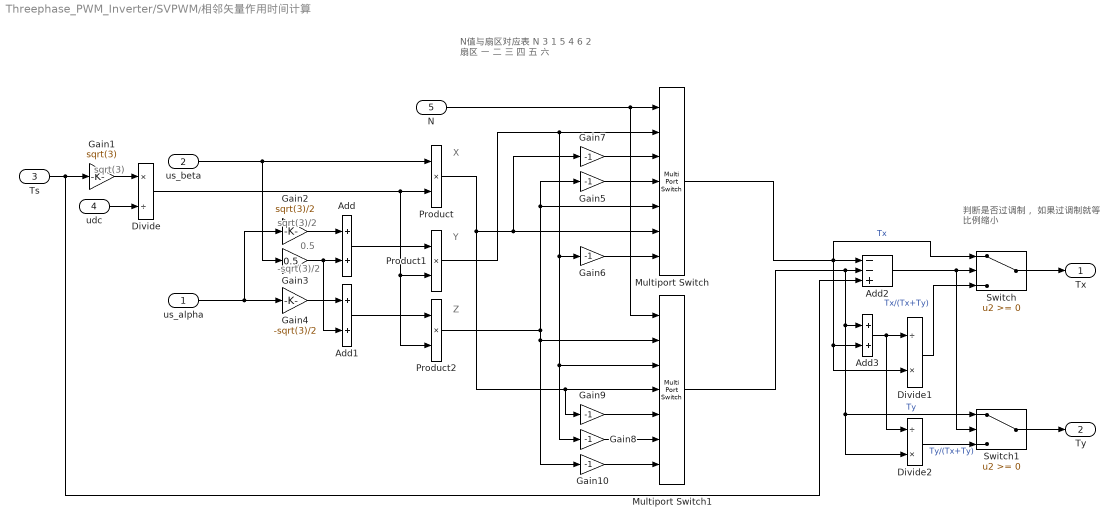
== system Threephase_PWM_Inverter/SVPWM/相邻矢量作用时间计算 ==
  note: 判断是否过调制，
      | 如果过调制就等
      | 比例缩小
  note: N值与扇区对应表
      | N         3    1    5    4    6    2
      | 扇区    一  二  三  四  五   六
  note: Z
  note: Y
  note: X
  note: 0.5
  note: sqrt(3)/2
  note: sqrt(3)
  note: -sqrt(3)/2
  us_alpha : Inport
  us_beta : Inport  Port=2
  Ts : Inport  Port=3
  udc : Inport  Port=4
  N : Inport  Port=5
  Add : Sum
  Add1 : Sum
  Add2 : Sum  Inputs=--+
  Add3 : Sum
  Divide : Product  Inputs=*/
  Divide1 : Product  Inputs=/*
  Divide2 : Product  Inputs=/*
  Gain1 : Gain  Gain=sqrt(3)
  Gain{5..10} (6 alike) : Gain  Gain=-1
  Gain2 : Gain  Gain=sqrt(3)/2
  Gain3 : Gain  Gain=0.5
  Gain4 : Gain  Gain=-sqrt(3)/2
  Multiport Switch : MultiPortSwitch  Inputs=6  SaturateOnIntegerOverflow=off  InputSameDT=off
  Multiport Switch1 : MultiPortSwitch  Inputs=6  SaturateOnIntegerOverflow=off  InputSameDT=off
  Product : Product
  Product1 : Product
  Product2 : Product
  Switch : Switch  SaturateOnIntegerOverflow=off  InputSameDT=off
  Switch1 : Switch  SaturateOnIntegerOverflow=off  InputSameDT=off
  Tx : Outport  VectorParamsAs1DForOutWhenUnconnected=off
  Ty : Outport  Port=2  VectorParamsAs1DForOutWhenUnconnected=off
  wires:
  Add1/1 -> Product2/1
  Ts/1 -> Add2/3, Gain1/1
  udc/1 -> Divide/2
  us_beta/1 -> Gain3/1, Product/1
  Gain5/1 -> Multiport Switch/4
  Gain1/1 -> Divide/1
  Product/1 -> Multiport Switch/6, Gain7/1, Gain9/1, Multiport Switch1/4
  Product1/1 -> Multiport Switch1/3, Gain8/1, Gain6/1, Multiport Switch/2
  us_alpha/1 -> Gain2/1, Gain4/1
  N/1 -> Multiport Switch1/1, Multiport Switch/1
  Gain9/1 -> Multiport Switch1/5
  Divide/1 -> Product2/2, Product1/2, Product/2
  Product2/1 -> Multiport Switch1/2, Gain10/1, Multiport Switch/5, Gain5/1
  Gain3/1 -> Add1/2, Add/2
  Gain6/1 -> Multiport Switch/7
  Gain7/1 -> Multiport Switch/3
  Gain4/1 -> Add1/1
  Gain8/1 -> Multiport Switch1/6
  Gain2/1 -> Add/1
  Add/1 -> Product1/1
  Gain10/1 -> Multiport Switch1/7
  Multiport Switch/1 -> Add3/2, Divide1/2, Switch/1, Add2/1  "Tx"
  Multiport Switch1/1 -> Divide2/2, Switch1/1, Add3/1, Add2/2  "Ty"
  Add2/1 -> Switch1/2, Switch/2
  Switch/1 -> Tx/1
  Add3/1 -> Divide2/1, Divide1/1
  Divide1/1 -> Switch/3  "Tx/(Tx+Ty)"
  Switch1/1 -> Ty/1
  Divide2/1 -> Switch1/3  "Ty/(Tx+Ty)"

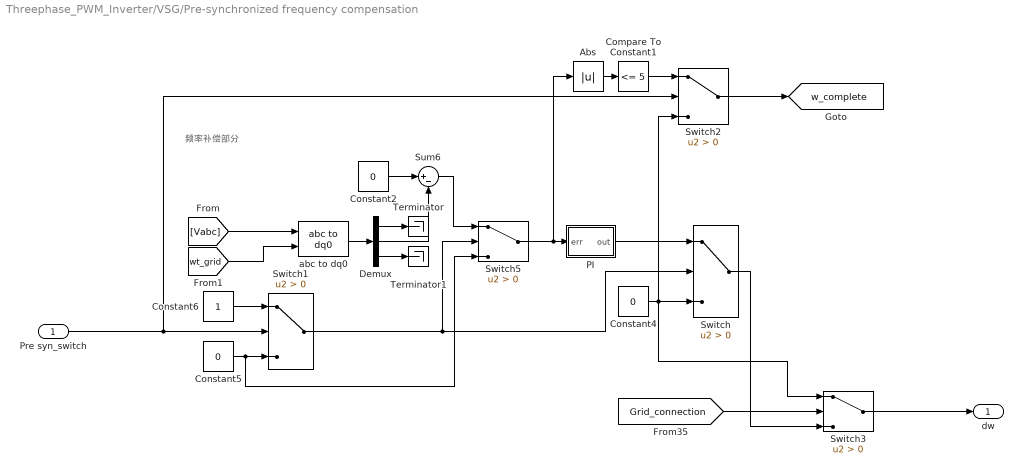
== system Threephase_PWM_Inverter/VSG/Pre-synchronized frequency compensation ==
  note: 频率补偿部分
  Pre syn_switch : Inport
  Abs : Abs  SaturateOnIntegerOverflow=off
  Compare To Constant1 : simulink/Logic and Bit Operations/Compare To Constant  relop=<=  const=5  OutDataTypeStr=boolean
  Constant2 : Constant  Value=0
  Constant4 : Constant  Value=0
  Constant5 : Constant  Value=0
  Constant6 : Constant
  Demux : Demux  Outputs=3
  PI : Subsystem
  Sum6 : Sum  Inputs=|+-
  Switch{,1..3,5} (5 alike) : Switch  Criteria=u2 > Threshold  SaturateOnIntegerOverflow=off  InputSameDT=off
  Terminator : Terminator
  Terminator1 : Terminator
  abc to dq0 : spsabctodq0Lib/abc to dq0  Alignment=90 degrees behind phase A axis
  dw : Outport  VectorParamsAs1DForOutWhenUnconnected=off
  tag scope: w_complete=global
  wires:
  Demux/2 -> Sum6/2
  Constant4/1 -> Switch/3, Switch3/1, Switch2/3
  Switch3/1 -> dw/1
  Switch/1 -> Switch3/3
  Pre syn_switch/1 -> Switch1/2, Switch2/2
  [wt_grid] -> abc to dq0/2
  Constant5/1 -> Switch1/3, Switch5/3
  Switch1/1 -> Switch/2, Switch5/2
  abc to dq0/1 -> Demux/1
  Constant2/1 -> Sum6/1
  [Vabc] -> abc to dq0/1
  Constant6/1 -> Switch1/1
  Switch5/1 -> Abs/1, PI/1(err)
  PI/1(out) -> Switch/1
  Sum6/1 -> Switch5/1
  Demux/1 -> Terminator/1
  Demux/3 -> Terminator1/1
  [Grid_connection] -> Switch3/2
  Switch2/1 -> [w_complete]
  Compare To Constant1/1 -> Switch2/1
  Abs/1 -> Compare To Constant1/1

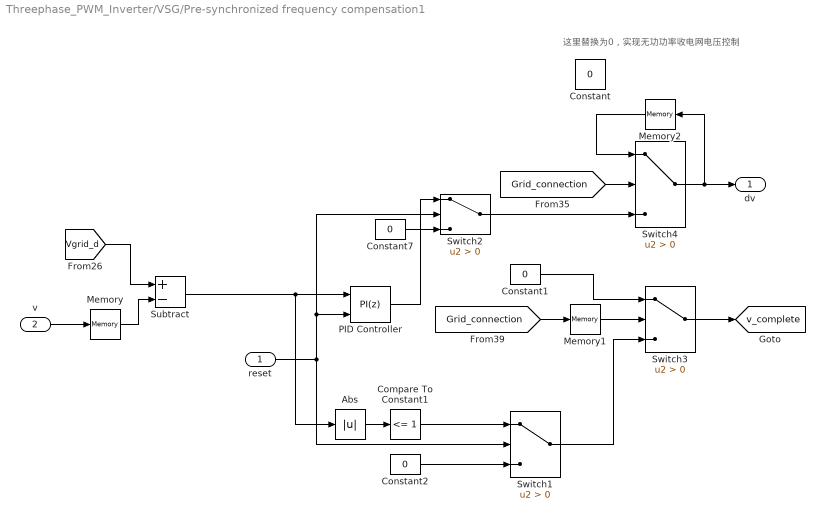
== system Threephase_PWM_Inverter/VSG/Pre-synchronized frequency compensation1 ==
  note: 这里替换为0，实现无功功率收电网电压控制
  reset : Inport
  v : Inport  Port=2
  Abs : Abs  SaturateOnIntegerOverflow=off
  Compare To Constant1 : simulink/Logic and Bit Operations/Compare To Constant  relop=<=  const=1  OutDataTypeStr=boolean
  Constant{,1..2,7} (4 alike) : Constant  Value=0
  Memory : Memory  InitialCondition=Vn
  Memory1 : Memory
  Memory2 : Memory
  PID Controller : slpidlib/PID Controller  Controller=PI  Form=Parallel  TimeDomain=Discrete-time  UseExternalTs=off  SampleTime=-1  IntegratorMethod=Forward Euler  FilterMethod=Forward Euler  ControllerParametersSource=internal  P=0.1  I=10  UseKiTs=off  D=0  N=100  UseFilter=on  TunerSelectOption=Transfer Function Based (PID Tuner App)  InitialConditionSource=internal  InitialConditionForIntegrator=0  InitialConditionForFilter=0  DifferentiatorICPrevScaledInput=0  ExternalReset=rising  TrackingMode=off  Kt=1  LimitOutput=on  SatLimitsSource=internal  UpperSaturationLimit=10  LowerSaturationLimit=-10  LinearizeAsGain=on  AntiWindupMode=none  Kb=1  LimitIntegrator=off  UpperIntegratorSaturationLimit=inf  LowerIntegratorSaturationLimit=-inf  POutMin=[]  POutMax=[]  IOutMin=[]  IOutMax=[]  DOutMin=[]  DOutMax=[]  NOutMin=[]  NOutMax=[]  SumOutMin=[]  SumOutMax=[]  SaturationOutMin=[]  SaturationOutMax=[]  PParamMin=[]  PParamMax=[]  IParamMin=[]  IParamMax=[]  DParamMin=[]  DParamMax=[]  NParamMin=[]  NParamMax=[]  KbParamMin=[]  KbParamMax=[]  KtParamMin=[]  KtParamMax=[]  KbOutMin=[]  KbOutMax=[]  KtOutMin=[]  KtOutMax=[]  IntegratorOutMin=[]  IntegratorOutMax=[]  FilterOutMin=[]  FilterOutMax=[]  SumI1OutMin=[]  SumI1OutMax=[]  SumI2OutMin=[]  SumI2OutMax=[]  SumI3OutMin=[]  SumI3OutMax=[]  SumI4OutMin=[]  SumI4OutMax=[]  SumDOutMin=[]  SumDOutMax=[]  DifferentiatorOutMin=[]  DifferentiatorOutMax=[]  FilterDiffOutCoefMin=[]  FilterDiffOutCoefMax=[]  ReciprocalOutMin=[]  ReciprocalOutMax=[]  SumDenOutMin=[]  SumDenOutMax=[]  SumNumOutMin=[]  SumNumOutMax=[]  DivideOutMin=[]  DivideOutMax=[]  UdiffTsProdOutMin=[]  UdiffTsProdOutMax=[]  NTsProdOutMin=[]  NTsProdOutMax=[]  UintegralTsProdOutMin=[]  UintegralTsProdOutMax=[]  UngainTsProdOutMin=[]  UngainTsProdOutMax=[]  ClampingZeroOutDataTypeStr=Inherit: Inherit via back propagation  ClampingZeroOutMin=[]  ClampingZeroOutMax=[]  FilterDenConstantOutDataTypeStr=Inherit: Inherit via back propagation  FilterDenConstantOutMin=[]  FilterDenConstantOutMax=[]  PCopyOutDataTypeStr=Inherit: Inherit via back propagation  PCopyOutMin=[]  PCopyOutMax=[]  NCopyOutDataTypeStr=Inherit: Inherit via back propagation  NCopyOutMin=[]  NCopyOutMax=[]  IntegratorContinuousStateAttributes=''  IntegratorStateMustResolveToSignalObject=off  IntegratorRTWStateStorageClass=Auto  FilterContinuousStateAttributes=''  FilterStateMustResolveToSignalObject=off  FilterRTWStateStorageClass=Auto  ParallelPVariant=InternalParameters  IdealPVariant=Disabled  IVariant=InternalParameters  DVariant=Disabled  IntegratorVariant=Discrete  SatVariant=Enabled  AWVariant=Passthrough  PCopyVariant=Disabled  TRVariant=Disabled  FdbkBlocksVariant=Forward  IdealPFdbkVariant=Disabled  SatFdbkVariant=Disabled  DerivativeFilterVariant=Disabled  NVariant=Disabled  NCopyVariant=Disabled_SignalSpec  FilterICVariant=Disabled  IntegratorICVariant=InternalICs  ExternalResetVariant=ExternalReset  TRSumVariant=Passthrough  SumFdbkVariant=Disabled  SumVariant=Sum_PI  TsampFilterVariant=InternalTs  TsampNgainVariant=Passthrough  TsampIntegralVariant=Passthrough  ExternalSaturationOutDataTypeStr=Inherit: Same as second input
  Subtract : Sum  Inputs=+-
  Switch{1..4} (4 alike) : Switch  Criteria=u2 > Threshold  SaturateOnIntegerOverflow=off  InputSameDT=off
  dv : Outport  VectorParamsAs1DForOutWhenUnconnected=off
  tag scope: v_complete=global
  wires:
  Switch4/1 -> dv/1, Memory2/1
  PID Controller/1 -> Switch2/1
  reset/1 -> PID Controller/2, Switch2/2, Switch1/2
  v/1 -> Memory/1
  Memory/1 -> Subtract/2
  Memory2/1 -> Switch4/1
  Constant7/1 -> Switch2/3
  Switch2/1 -> Switch4/3
  Subtract/1 -> PID Controller/1, Abs/1
  [Vgrid_d] -> Subtract/1
  [Grid_connection] -> Switch4/2
  Compare To Constant1/1 -> Switch1/1
  Abs/1 -> Compare To Constant1/1
  [Grid_connection] -> Memory1/1
  Memory1/1 -> Switch3/2
  Switch1/1 -> Switch3/3
  Switch3/1 -> [v_complete]
  Constant1/1 -> Switch3/1
  Constant2/1 -> Switch1/3

== system Threephase_PWM_Inverter/VSG/Pre-synchronized frequency compensation/PI ==
  err : Inport
  Add : Sum
  Gain1 : Gain  Gain=10
  Gain3 : Gain  Gain=0.1
  Integrator : Integrator  LimitOutput=on  UpperSaturationLimit=10  LowerSaturationLimit=-10
  Saturation : Saturate  UpperLimit=6  LowerLimit=-6
  out : Outport  VectorParamsAs1DForOutWhenUnconnected=off
  wires:
  err/1 -> Gain1/1, Gain3/1
  Gain1/1 -> Integrator/1
  Gain3/1 -> Add/1
  Integrator/1 -> Add/2
  Add/1 -> Saturation/1
  Saturation/1 -> out/1
